simulink model "quadXYsim"  (R2018b)
settings: Solver=FixedStepAuto  StartTime=0.0  StopTime=tfinal  FixedStep=dt  RelTol=1e-3
values from neighbouring files (symbols this model uses):
  Kdpsi = 0.067644*1    (= 0.067644)    [quadSimRunMain.m]
  Kipsi = 0.045028*.0    (= 0)    [quadSimRunMain.m]
  Kppsi = 0.11038*1    (= 0.11038)    [quadSimRunMain.m]
  Npsi = 1/Tfpsi    (= 159.182438993)    [quadSimRunMain.m]
  param = quadparam    [quadDyn.m]    (also in quadDynSimple.m; quadSimRunMain.m; quadcomputeFandT.m; quadcomputeMotorSpeed.m)
  Upsisat = 100*param.m*param.g(3)*0.1    [quadSimRunMain.m]
libraries: simulink x2
settings Model: Creator=duho46  LastModifiedBy=duho46

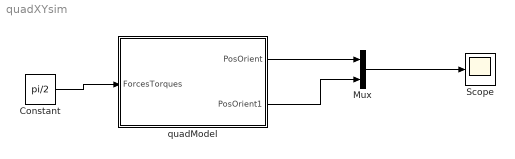
== system quadXYsim ==
  Constant : Constant  Value=pi/2
  Mux : Mux  Inputs=2
  Scope : Scope
  quadModel : Subsystem
      mask Display: image('C:\Users\duho46\Pictures\3D Robotics Solo.jpg');
  wires:
  Constant/1 -> quadModel/1(ForcesTorques)
  quadModel/1(PosOrient) -> Mux/1
  quadModel/2(PosOrient1) -> Mux/2
  Mux/1 -> Scope/1

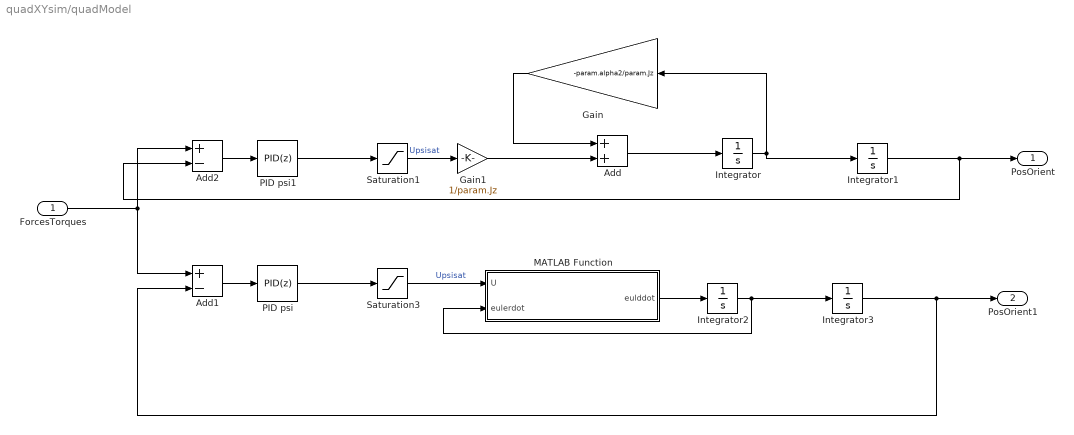
== system quadXYsim/quadModel ==
  ForcesTorques : Inport
  Add : Sum
  Add1 : Sum  Inputs=+-
  Add2 : Sum  Inputs=+-
  Gain : Gain  Gain=-param.alpha2/param.Jz
  Gain1 : Gain  Gain=1/param.Jz
  Integrator{,1..3} (4 alike) : Integrator
  MATLAB Function : MATLAB Function  TreatAsAtomicUnit=on
  PID psi : simulink/Continuous/PID Controller  Controller=PID  Form=Parallel  TimeDomain=Discrete-time  SampleTime=-1  IntegratorMethod=Forward Euler  FilterMethod=Forward Euler  ControllerParametersSource=internal  P=Kppsi  I=Kipsi  D=Kdpsi  UseFilter=off  N=Npsi  TunerSelectOption=Transfer Function Based (PID Tuner App)  InitialConditionSource=internal  InitialConditionForIntegrator=0  InitialConditionForFilter=0  DifferentiatorICPrevScaledInput=0  ExternalReset=none  TrackingMode=off  Kt=1  LimitOutput=off  UpperSaturationLimit=inf  LowerSaturationLimit=-inf  LinearizeAsGain=on  AntiWindupMode=none  Kb=1  POutMin=[]  POutMax=[]  IOutMin=[]  IOutMax=[]  DOutMin=[]  DOutMax=[]  NOutMin=[]  NOutMax=[]  SumOutMin=[]  SumOutMax=[]  SaturationOutMin=[]  SaturationOutMax=[]  PParamMin=[]  PParamMax=[]  IParamMin=[]  IParamMax=[]  DParamMin=[]  DParamMax=[]  NParamMin=[]  NParamMax=[]  KbParamMin=[]  KbParamMax=[]  KtParamMin=[]  KtParamMax=[]  KbOutMin=[]  KbOutMax=[]  KtOutMin=[]  KtOutMax=[]  IntegratorOutMin=[]  IntegratorOutMax=[]  FilterOutMin=[]  FilterOutMax=[]  SumI1OutMin=[]  SumI1OutMax=[]  SumI2OutMin=[]  SumI2OutMax=[]  SumI3OutMin=[]  SumI3OutMax=[]  SumI4OutMin=[]  SumI4OutMax=[]  SumDOutMin=[]  SumDOutMax=[]  DifferentiatorOutMin=[]  DifferentiatorOutMax=[]  FilterDiffOutCoefMin=[]  FilterDiffOutCoefMax=[]  ReciprocalOutMin=[]  ReciprocalOutMax=[]  SumDenOutMin=[]  SumDenOutMax=[]  SumNumOutMin=[]  SumNumOutMax=[]  DivideOutMin=[]  DivideOutMax=[]  IntegratorContinuousStateAttributes=''  IntegratorStateMustResolveToSignalObject=off  IntegratorRTWStateStorageClass=Auto  FilterContinuousStateAttributes=''  FilterStateMustResolveToSignalObject=off  FilterRTWStateStorageClass=Auto  ParallelPVariant=InternalParameters  IdealPVariant=Disabled  IVariant=InternalParameters  DVariant=InternalParameters  IntegratorVariant=Discrete  SatVariant=Disabled  AWVariant=Passthrough  PCopyVariant=Disabled  TRVariant=Disabled  FdbkBlocksVariant=Forward  IdealPFdbkVariant=Disabled  SatFdbkVariant=Disabled  DerivativeFilterVariant=Differentiator  NVariant=Passthrough  NCopyVariant=Disabled_SignalSpec  FilterICVariant=InternalICsDifferentiator  IntegratorICVariant=InternalICs  ExternalResetVariant=Disabled  TRSumVariant=Passthrough  SumFdbkVariant=Disabled  SumVariant=Sum_PID
  PID psi1 : simulink/Continuous/PID Controller  Controller=PID  Form=Parallel  TimeDomain=Discrete-time  SampleTime=-1  IntegratorMethod=Forward Euler  FilterMethod=Forward Euler  ControllerParametersSource=internal  P=Kppsi  I=Kipsi  D=Kdpsi  UseFilter=off  N=Npsi  TunerSelectOption=Transfer Function Based (PID Tuner App)  InitialConditionSource=internal  InitialConditionForIntegrator=0  InitialConditionForFilter=0  DifferentiatorICPrevScaledInput=0  ExternalReset=none  TrackingMode=off  Kt=1  LimitOutput=off  UpperSaturationLimit=inf  LowerSaturationLimit=-inf  LinearizeAsGain=on  AntiWindupMode=none  Kb=1  POutMin=[]  POutMax=[]  IOutMin=[]  IOutMax=[]  DOutMin=[]  DOutMax=[]  NOutMin=[]  NOutMax=[]  SumOutMin=[]  SumOutMax=[]  SaturationOutMin=[]  SaturationOutMax=[]  PParamMin=[]  PParamMax=[]  IParamMin=[]  IParamMax=[]  DParamMin=[]  DParamMax=[]  NParamMin=[]  NParamMax=[]  KbParamMin=[]  KbParamMax=[]  KtParamMin=[]  KtParamMax=[]  KbOutMin=[]  KbOutMax=[]  KtOutMin=[]  KtOutMax=[]  IntegratorOutMin=[]  IntegratorOutMax=[]  FilterOutMin=[]  FilterOutMax=[]  SumI1OutMin=[]  SumI1OutMax=[]  SumI2OutMin=[]  SumI2OutMax=[]  SumI3OutMin=[]  SumI3OutMax=[]  SumI4OutMin=[]  SumI4OutMax=[]  SumDOutMin=[]  SumDOutMax=[]  DifferentiatorOutMin=[]  DifferentiatorOutMax=[]  FilterDiffOutCoefMin=[]  FilterDiffOutCoefMax=[]  ReciprocalOutMin=[]  ReciprocalOutMax=[]  SumDenOutMin=[]  SumDenOutMax=[]  SumNumOutMin=[]  SumNumOutMax=[]  DivideOutMin=[]  DivideOutMax=[]  IntegratorContinuousStateAttributes=''  IntegratorStateMustResolveToSignalObject=off  IntegratorRTWStateStorageClass=Auto  FilterContinuousStateAttributes=''  FilterStateMustResolveToSignalObject=off  FilterRTWStateStorageClass=Auto  ParallelPVariant=InternalParameters  IdealPVariant=Disabled  IVariant=InternalParameters  DVariant=InternalParameters  IntegratorVariant=Discrete  SatVariant=Disabled  AWVariant=Passthrough  PCopyVariant=Disabled  TRVariant=Disabled  FdbkBlocksVariant=Forward  IdealPFdbkVariant=Disabled  SatFdbkVariant=Disabled  DerivativeFilterVariant=Differentiator  NVariant=Passthrough  NCopyVariant=Disabled_SignalSpec  FilterICVariant=InternalICsDifferentiator  IntegratorICVariant=InternalICs  ExternalResetVariant=Disabled  TRSumVariant=Passthrough  SumFdbkVariant=Disabled  SumVariant=Sum_PID
  Saturation1 : Saturate  UpperLimit=Upsisat  LowerLimit=-Upsisat
  Saturation3 : Saturate  UpperLimit=Upsisat  LowerLimit=-Upsisat
  PosOrient : Outport
  PosOrient1 : Outport  Port=2
  wires:
  Gain/1 -> Add/1
  Gain1/1 -> Add/2
  Add/1 -> Integrator/1
  Integrator/1 -> Gain/1, Integrator1/1
  MATLAB Function/1(eulddot) -> Integrator2/1
  Integrator2/1 -> Integrator3/1, MATLAB Function/2(eulerdot)
  Integrator3/1 -> Add1/2, PosOrient1/1
  Integrator1/1 -> Add2/2, PosOrient/1
  PID psi/1 -> Saturation3/1
  Saturation3/1 -> MATLAB Function/1(U)  "Upsisat"
  ForcesTorques/1 -> Add1/1, Add2/1
  Add1/1 -> PID psi/1
  Add2/1 -> PID psi1/1
  PID psi1/1 -> Saturation1/1
  Saturation1/1 -> Gain1/1  "Upsisat"

== matlab function quadXYsim/quadModel/MATLAB Function ==
  data: U input; eulddot output; eulerdot input
function eulddot = fcn(U,eulerdot)

param.m = 0.5;
param.g = [0 0 9.81]';
param.cd = 0.32;
param.cf = 1e-4;
param.L = 0.5;
param.ct = 1e-5;
param.Jx = 0.002;
param.Jy = 0.002;
param.Jz = 0.003;
param.lambda1 = 0.36;
param.lambda2 = 0.6;
param.alpha1 = 0.002;
param.alpha2 = 0.005;

eulddot = U/param.Jz - param.alpha2*eulerdot/param.Jz;
